simulink model "bai29"  (R2021b)
settings: Solver=VariableStepAuto  StartTime=0.0  StopTime=10.0  RelTol=1e-3  EnableMultiTasking=on
settings Model: Creator=Dell  LastModifiedBy=Leon8dem1god
settings SolverCC: AlgebraicLoopSolver=TrustRegion
settings DataIOCC: ReturnWorkspaceOutputs=off
settings OptimizationCC: LifeSpan=inf
settings DebuggingCC: SFUnexpectedBacktrackingDiag=warning  SFNoUnconditionalDefaultTransitionDiag=warning  SFMachineParentedDataDiag=warning  ArithmeticOperatorsInVariantConditions=warning
settings SFSimCC: SimUseLocalCustomCode=off  CustomCodeUndefinedFunction=UseInterfaceOnly
settings RTWCC: RTWUseLocalCustomCode=off
settings CodeAppCC: StateflowObjectComments=on
settings GRTTargetCC: TargetLangStandard=C89/C90 (ANSI)
settings ConfigComp: CovMetricSettings=dw  CovSaveCumulativeToWorkspaceVar=on  CovSaveSingleToWorkspaceVar=on  CovExternalEMLEnable=off

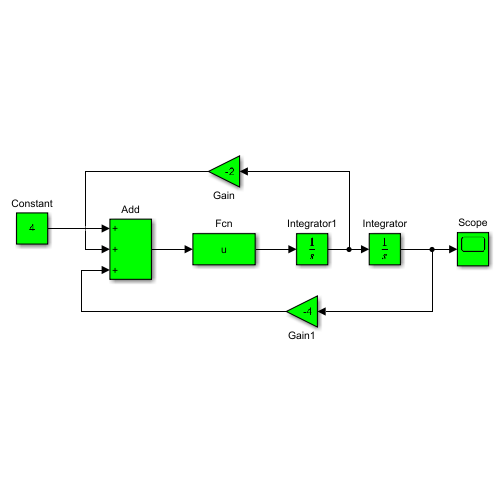
[thumbnail: Simulink's stored preview of the top-level diagram]
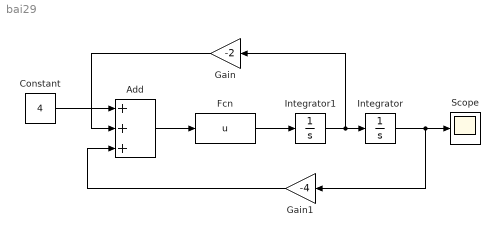
== system bai29 ==
  Add : Sum  Inputs=+++
  Constant : Constant  Value=4
  Fcn : Fcn  Expr=u
  Gain : Gain  Gain=-2
  Gain1 : Gain  Gain=-4
  Integrator : Integrator  InitialCondition=1
  Integrator1 : Integrator  InitialCondition=1
  Scope : Scope
  wires:
  Gain1/1 -> Add/3
  Gain/1 -> Add/2
  Add/1 -> Fcn/1
  Fcn/1 -> Integrator1/1
  Integrator1/1 -> Gain/1, Integrator/1
  Constant/1 -> Add/1
  Integrator/1 -> Scope/1, Gain1/1
